simulink model "HolonomicSimulator"  (Simulink 7.5)
settings: Solver=ode45  StartTime=0.0  StopTime=20  RelTol=1e-3
values from neighbouring files (symbols this model uses):
  A = [zeros(3,3),eye(3,3);zeros(3,6)]    [LQRHolonomic.m]
  B = [zeros(3,4);0 -1 0 1;1 0 -1 0;Ra Ra Ra Ra]    [LQRHolonomic.m]
undefined symbols (not defined in the file or in its folder): K
libraries: mblibv1 x10, simulink x2
settings Model: Creator=Edoardo  LastModifiedBy=Edoardo

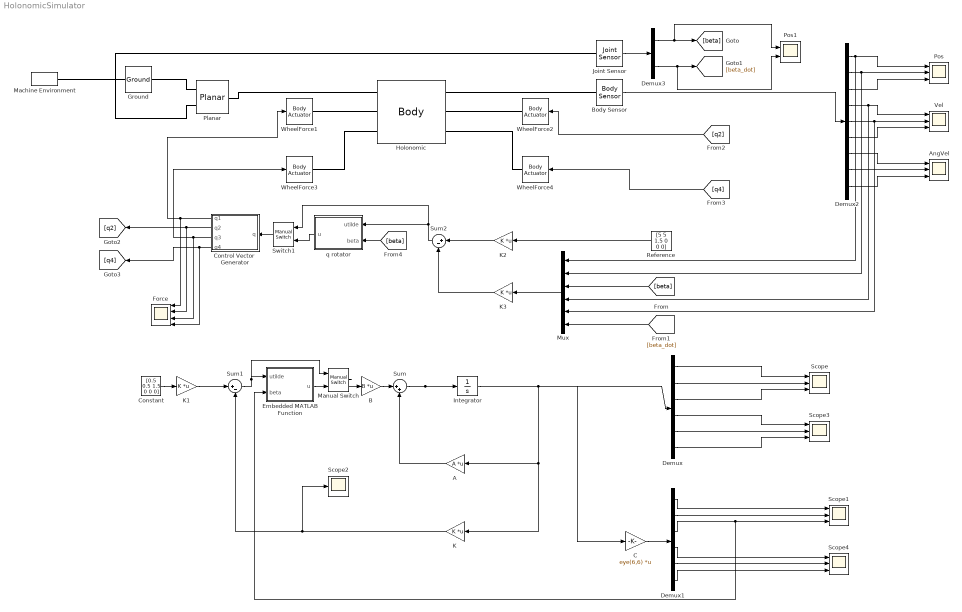
== system HolonomicSimulator ==
  A : Gain  Gain=A  Multiplication=Matrix(K*u)  ParameterDataType=fixdt(1, 16)  ParameterScaling=2^0  OutDataType=fixdt(1, 16)  OutScaling=2^0
  AngVel : Scope  NumInputPorts=3
      settings: YMin=-5~-5~-5  YMax=5~5~5  SaveName=ScopeData7
  B : Gain  Gain=B  Multiplication=Matrix(K*u)  ParameterDataType=fixdt(1, 16)  ParameterScaling=2^0  OutDataType=fixdt(1, 16)  OutScaling=2^0
  Body Sensor : mblibv1/Sensors &  Actuators/Body Sensor  DialogController=MECH.DynMechDlgSource  SystemSampleTime=-1  UpdateFromCAD=off  PhysicalDomain=Mechanical  PortType=blob  Muxed=on  Pose=off  Angle=on  AngleUnits=deg  ArcVelocity=on  ArcVelocityUnits=rad/s  ArcAcceleration=off  ArcAccelerationUnits=deg/s^2  CoordPosition=on  CoordPositionUnits=m  Velocity=on  VelocityUnits=m/s  Acceleration=off  AccelerationUnits=m/s^2  Quaternion=on  QuaternionDT=off  QuaternionDDT=off  QuaternionUnits=off  OutputVector=[1]  ActiveIO=on  Width=9  DialogClass=MechanicalSensorBlock  ReferenceFrame=Absolute (World)
  C : Gain  Gain=eye(6,6)  Multiplication=Matrix(K*u)  ParameterDataType=fixdt(1, 16)  ParameterScaling=2^0  OutDataType=fixdt(1, 16)  OutScaling=2^0
  Constant : Constant  Value=[0.5 0.5 1.5 0 0 0]  OutDataType=fixdt(1, 16)  OutScaling=2^0
  Control Vector  Generator : Stateflow chart  TreatAsAtomicUnit=on
  Demux : Demux  Outputs=6
  Demux1 : Demux  Outputs=6
  Demux2 : Demux  Outputs=9
  Demux3 : Demux  Outputs=2
  Embedded MATLAB Function : Stateflow chart  TreatAsAtomicUnit=on
  Force : Scope  NumInputPorts=4
      settings: YMin=-5~-5~-5~-5  YMax=5~5~5~5  SaveName=ScopeData9
  Ground : mblibv1/Bodies/Ground  DialogController=MECH.DynMechDlgSource  SystemSampleTime=-1  UpdateFromCAD=off  LeftPortType=env  RightPortType=workingframe  PhysicalDomain=Mechanical  DialogClass=GroundBlock  CoordPosition=[0 0 0]  CoordPositionUnits=m  StateVectorMgrId=0  MachineId=[1 0]  ShowEnvPort=on
  Holonomic : mblibv1/Bodies/Body  DialogController=MECH.DynMechDlgSource  PhysicalDomain=mechanical  SubClassName=Unknown  LeftPortType=workingframe  RightPortType=workingframe  LConnTagsString=CG|CS1|CS3  RConnTagsString=CS5|CS2|CS4  UpdateFromCAD=off  DialogClass=MechanicalBodyBlock  Mass=4.3  MassUnits=kg  InertiaUnits=kg*m^2  Inertia=[0.1 0 0;0 0.1 0; 0 0 0.0505]  Shape=Cylinder  ShapeDims=[1 1]  ShapeUnits=m  ShapeUse=false  Density=1  DensityUnits=kg/m^3  DensityUse=false  GraphicsMode=MACHINE_DEFAULT  BodyColorSelMode=MACHINE_DEFAULT  BodyColor=[1 0 0]  AttachedToCS=CG  CG=Left$CG$[0 0 0]$WORLD$WORLD$m$[0 0 0]$Euler X-Y-Z$deg$WORLD$true$none  WorkingFrames=Right$CS5$[0 0 0]$CG$CG$m$[0 0 0]$Euler X-Y-Z$deg$WORLD$true$none#Left$CS1$[0.155 0 0]$CG$CG$m$[0 0 0]$Euler X-Y-Z$deg$WORLD$true$none#Right$CS2$[0 0.155 0]$CG$CG$m$[0 0 0]$Euler X-Y-Z$deg$WORLD$true$none#Right$CS4$[0 -0.155 0]$CG$CG$m$[0 0 0]$Euler X-Y-Z$deg$WORLD$true$none#Left$CS3$[-0.155 0 0]$CG$CG$m$[0 0 0]$Euler X-Y-Z$deg$WORLD$true$none  CGPos=[0 0 0]  CGRot=[0 0 0]  CS0Pos=[]  CS0Rot=[]  CS1Pos=[0.155 0 0]  CS1Rot=[0 0 0]  CS2Pos=[0 0.155 0]  CS2Rot=[0 0 0]  CS3Pos=[-0.155 0 0]  CS3Rot=[0 0 0]  CS4Pos=[0 -0.155 0]  CS4Rot=[0 0 0]  CS5Pos=[0 0 0]  CS5Rot=[0 0 0]  CS6Pos=[]  CS6Rot=[]  CS7Pos=[]  CS7Rot=[]  CS8Pos=[]  CS8Rot=[]  CS9Pos=[]  CS9Rot=[]  CS10Pos=[]  CS10Rot=[]  CS11Pos=[]  CS11Rot=[]  CS12Pos=[]  CS12Rot=[]  CS13Pos=[]  CS13Rot=[]  CS14Pos=[]  CS14Rot=[]  CS15Pos=[]  CS15Rot=[]  CS16Pos=[]  CS16Rot=[]  CS17Pos=[]  CS17Rot=[]  CS18Pos=[]  CS18Rot=[]  CS19Pos=[]  CS19Rot=[]  CS20Pos=[]  CS20Rot=[]
  Integrator : Integrator  InitialCondition=[0 0 0 0 0 0]
  Joint Sensor : mblibv1/Sensors &  Actuators/Joint Sensor  DialogController=MECH.DynMechDlgSource  SystemSampleTime=-1  UpdateFromCAD=off  PhysicalDomain=Mechanical  PortType=blob  Muxed=on  Pose=off  Angle=on  AngleUnits=rad  ArcVelocity=on  ArcVelocityUnits=rad/s  ArcAcceleration=off  ArcAccelerationUnits=deg/s^2  CoordPosition=off  CoordPositionUnits=m  Velocity=off  VelocityUnits=m/s  Acceleration=off  AccelerationUnits=m/s^2  Quaternion=on  QuaternionDT=off  QuaternionDDT=off  QuaternionUnits=off  OutputVector=[1]  ActiveIO=on  Width=2  DialogClass=MechanicalSensorBlock  Primitive=R1  Force=off  ForceUnits=N  Torque=off  TorqueUnits=N*m  ReferenceFrame=Absolute (World)  ReactionSensedSide=Follower  ReactionReferenceFrame=Absolute (World)  ReactionForce=off  ReactionForceUnits=N  ReactionMoment=off  ReactionMomentUnits=N*m
  K : Gain  Gain=K  Multiplication=Matrix(K*u)  ParameterDataType=fixdt(1, 16)  ParameterScaling=2^0  OutDataType=fixdt(1, 16)  OutScaling=2^0
  K1 : Gain  Gain=K  Multiplication=Matrix(K*u)  ParameterDataType=fixdt(1, 16)  ParameterScaling=2^0  OutDataType=fixdt(1, 16)  OutScaling=2^0
  K2 : Gain  Gain=K  Multiplication=Matrix(K*u) (u vector)  ParameterDataType=fixdt(1, 16)  ParameterScaling=2^0  OutDataType=fixdt(1, 16)  OutScaling=2^0
  K3 : Gain  Gain=K  Multiplication=Matrix(K*u) (u vector)  ParameterDataType=fixdt(1, 16)  ParameterScaling=2^0  OutDataType=fixdt(1, 16)  OutScaling=2^0
  Machine Environment : mblibv1/Bodies/Machine Environment  DialogController=MECH.DialogSource  SystemSampleTime=-1  PortType=env  PhysicalDomain=Mechanical  DialogTemplateClass=MECH.MachineEnvironment  SyncWhenCopied=off  Gravity=[0 0 -9.81]  GravityUnits=m/s^2  GravityAsSignal=off  Dimensionality=Auto-detect  AnalysisType=Forward dynamics  LinearAssemblyTolerance=1e-3  LinearAssemblyToleranceUnits=m  AngularAssemblyTolerance=1e-3  AngularAssemblyToleranceUnits=rad  ConstraintSolverType=Stabilizing  ConstraintRelTolerance=1e-4  ConstraintAbsTolerance=1e-4  UseRobustSingularityHandling=off  RedundancyAnalysisToleranceType=Automatically select tolerance  RedundancyAnalysisTolerance=1e-14  StatePerturbationType=Fixed  PerturbationSize=1e-5  VisualizeMachine=on  BodyVisualizationType=Use model default body geometries  BodyColorSelMode=Use model default  DefaultBodyColor=[1 0 0]
  Manual Switch : simulink/Signal Routing/Manual Switch  SystemSampleTime=-1  sw=1  action=0  varsize=off
  Mux : Mux  Inputs=6
  Planar : mblibv1/Joints/Planar  DialogController=MECH.DynMechDlgSource  PhysicalDomain=mechanical  SubClassName=Unknown  LeftPortType=blob  RightPortType=blob  LConnTagsString=__newl0|SA1  RConnTagsString=__newr0  UpdateFromCAD=off  NumSAPorts=1  CutJoint=off  MarkAsCut=off  Primitives=prismatic_prismatic  PrimitiveProps=P1$World$[1 0 0]$prismatic#P2$World$[0 1 0]$prismatic#R1$World$[0 0 1]$revolute  DialogClass=JointBlock  P1Axis=[1 0 0]  P2Axis=[0 1 0]  R1Axis=[0 0 1]
  Pos : Scope  NumInputPorts=3
      settings: YMin=-5~-5~-5  YMax=5~5~5  SaveName=ScopeData5  MaxDataPoints=20000
  Pos1 : Scope  NumInputPorts=2
      settings: YMin=-5~-5  YMax=5~5  SaveName=ScopeData8  MaxDataPoints=15000
  Reference : Constant  Value=[5 5 1.5 0 0 0]  OutDataType=fixdt(1, 16)  OutScaling=2^0
  Scope{,1,3..4} (4 alike) : Scope  NumInputPorts=3
      Scope settings: YMin=-5~-5~-5  YMax=5~5~5
      Scope1 settings: YMin=-5~-5~-5  YMax=5~5~5
      Scope3 settings: YMin=-5~-5~-5  YMax=5~5~5  SaveName=ScopeData3
      Scope4 settings: YMin=-5~-5~-5  YMax=5~5~5  SaveName=ScopeData4
  Scope2 : Scope
      settings: SaveName=ScopeData2
  Sum : Sum  Inputs=|++  OutDataType=fixdt(1, 16)  OutScaling=2^0
  Sum1 : Sum  Inputs=|+-  OutDataType=fixdt(1, 16)  OutScaling=2^0
  Sum2 : Sum  Inputs=|+-  OutDataType=fixdt(1, 16)  OutScaling=2^0
  Switch1 : simulink/Signal Routing/Manual Switch  SystemSampleTime=-1  sw=0  action=0  varsize=off
  Vel : Scope  NumInputPorts=3
      settings: YMin=-5~-5~-5  YMax=5~5~5  SaveName=ScopeData6
  WheelForce{1..4} (4 alike) : mblibv1/Sensors &  Actuators/Body Actuator  DialogController=MECH.DynMechDlgSource  SystemSampleTime=-1  UpdateFromCAD=off  PhysicalDomain=Mechanical  PortType=blob  ActuationStyle=Force  AngleUnits=deg  ArcVelocityUnits=deg/s  ArcAccelerationUnits=deg/s^2  CoordPositionUnits=m  VelocityUnits=m/s  AccelerationUnits=m/s^2  ForceUnits=N  TorqueUnits=N*m  ActiveIO=on  Width=3  DialogClass=MechanicalActuatorBlock  ReferenceFrame=Local (Body CS)  Angle=off  CoordPosition=on  Force=on  Torque=off
  q rotator : Stateflow chart  TreatAsAtomicUnit=on
  wires:
  B/1 -> Sum/1
  A/1 -> Sum/2
  Integrator/1 -> A/1, K/1, C/1
  Sum/1 -> Integrator/1, Demux/1
  K1/1 -> Sum1/1
  K/1 -> Sum1/2, Scope2/1
  Constant/1 -> K1/1
  C/1 -> Demux1/1
  Demux/1 -> Scope/1
  Demux/2 -> Scope/2
  Demux/4 -> Scope3/1
  Demux/5 -> Scope3/2
  Demux/6 -> Scope3/3
  Demux1/1 -> Scope1/1
  Demux1/2 -> Scope1/2
  Demux1/3 -> Scope1/3, Embedded MATLAB Function/2(beta)
  Demux1/4 -> Scope4/1
  Demux1/5 -> Scope4/2
  Demux1/6 -> Scope4/3
  Demux/3 -> Scope/3
  Sum1/1 -> Embedded MATLAB Function/1(utilde), Manual Switch/1
  Manual Switch/1 -> B/1
  Embedded MATLAB Function/1(u) -> Manual Switch/2
  Demux2/1 -> Pos/1, Mux/1
  Demux2/2 -> Pos/2, Mux/2
  Demux2/4 -> Vel/1, Mux/4
  Demux2/5 -> Vel/2, Mux/5
  Demux2/6 -> Vel/3
  Demux2/3 -> Pos/3
  Body Sensor/1 -> Demux2/1
  Reference/1 -> K2/1
  Demux2/7 -> AngVel/1
  Demux2/8 -> AngVel/2
  Demux2/9 -> AngVel/3
  Mux/1 -> K3/1
  Joint Sensor/1 -> Demux3/1
  Demux3/1 -> [beta], Pos1/1
  Demux3/2 -> [beta_dot], Pos1/2
  [beta] -> Mux/3
  [beta_dot] -> Mux/6
  K2/1 -> Sum2/1
  K3/1 -> Sum2/2
  Control Vector  Generator/1(q1) -> WheelForce1/1, Force/1
  Control Vector  Generator/2(q2) -> [q2], Force/2
  Control Vector  Generator/3(q3) -> WheelForce3/1, Force/3
  Control Vector  Generator/4(q4) -> [q4], Force/4
  [q2] -> WheelForce2/1
  [q4] -> WheelForce4/1
  Sum2/1 -> q rotator/1(utilde), Switch1/1
  [beta] -> q rotator/2(beta)
  Switch1/1 -> Control Vector  Generator/1(q)
  q rotator/1(u) -> Switch1/2
  connections:
  Ground/RConn1 -- Planar/LConn1
  Planar/RConn1 -- Holonomic/LConn1
  Holonomic/LConn2 -- WheelForce1/RConn1
  WheelForce3/RConn1 -- Holonomic/LConn3
  Holonomic/RConn2 -- WheelForce2/RConn1
  WheelForce4/RConn1 -- Holonomic/RConn3
  Body Sensor/LConn1 -- Holonomic/RConn1
  Joint Sensor/LConn1 -- Planar/LConn2
  Machine Environment/RConn1 -- Ground/LConn1

== matlab function Control Vector Generator ==
  data: q1 output double; q input double; q2 output double; q3 output double; q4 output double
function [q1,q2,q3,q4] = fcn(q)
%#eml
q1=[0,q(1),0];
q2=[-q(2),0,0];
q3=[0,-q(3),0];
q4=[q(4),0,0];

== matlab function Embedded MATLAB Function ==
  data: u output double; utilde input double; beta input double
function u = fcn(utilde,beta)
%#eml
coth=cos(beta);
sith=sin(beta);
Rot=[ (coth^2/2 + coth/2 + sith^2/2)/(coth^2 + sith^2),                       sith/(2*(coth^2 + sith^2)), (coth^2/2 - coth/2 + sith^2/2)/(coth^2 + sith^2),                      -sith/(2*(coth^2 + sith^2));
                      -sith/(2*(coth^2 + sith^2)), (coth^2/2 + coth/2 + sith^2/2)/(coth^2 + sith^2),                       sith/(2*(coth^2 + sith^2)), (coth^2/2 - coth/2 + sith^2/2)/(coth^2 + sith^2);
 (coth^2/2 - coth/2 + sith^2/2)/(coth^2 + sith^2),                      -sith/(2*(coth^2 + sith^2)), (coth^2/2 + coth/2 + sith^2/2)/(coth^2 + sith^2),                       sith/(2*(coth^2 + sith^2));
                       sith/(2*(coth^2 + sith^2)), (coth^2/2 - coth/2 + sith^2/2)/(coth^2 + sith^2),                      -sith/(2*(coth^2 + sith^2)), (coth^2/2 + coth/2 + sith^2/2)/(coth^2 + sith^2)];
 
u =Rot*utilde;

== matlab function q rotator ==
  data: u output double; utilde input double; beta input double
function u = fcn(utilde,beta)
%#eml
coth=cos(beta);
sith=sin(beta);
Rot=[ (coth^2/2 + coth/2 + sith^2/2)/(coth^2 + sith^2),                       sith/(2*(coth^2 + sith^2)), (coth^2/2 - coth/2 + sith^2/2)/(coth^2 + sith^2),                      -sith/(2*(coth^2 + sith^2));
                      -sith/(2*(coth^2 + sith^2)), (coth^2/2 + coth/2 + sith^2/2)/(coth^2 + sith^2),                       sith/(2*(coth^2 + sith^2)), (coth^2/2 - coth/2 + sith^2/2)/(coth^2 + sith^2);
 (coth^2/2 - coth/2 + sith^2/2)/(coth^2 + sith^2),                      -sith/(2*(coth^2 + sith^2)), (coth^2/2 + coth/2 + sith^2/2)/(coth^2 + sith^2),                       sith/(2*(coth^2 + sith^2));
                       sith/(2*(coth^2 + sith^2)), (coth^2/2 - coth/2 + sith^2/2)/(coth^2 + sith^2),                      -sith/(2*(coth^2 + sith^2)), (coth^2/2 + coth/2 + sith^2/2)/(coth^2 + sith^2)];
 
u =Rot*utilde;
